simulink model "part7LQR"  (R2022a)
settings: Solver=VariableStepAuto  StartTime=0.0  StopTime=10.0  RelTol=1e-3
settings Model: Creator=HP  LastModifiedBy=HP

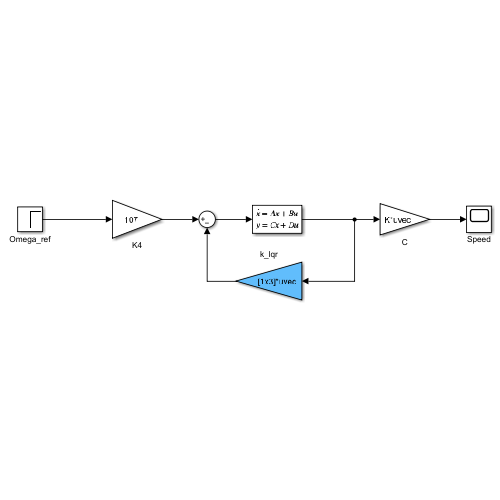
[thumbnail: Simulink's stored preview of the top-level diagram]
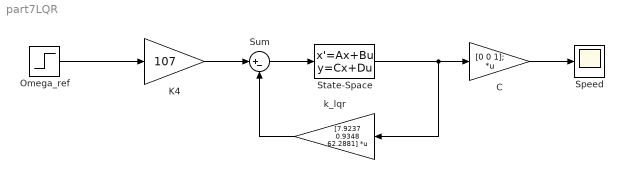
== system part7LQR ==
  C : Gain  Gain=[0 0 1];  Multiplication=Matrix(K*u) (u vector)
  K4 : Gain  Gain=107
  Omega_ref : Step  Time=0  SampleTime=0
  Speed : Scope
  State-Space : StateSpace  A=[-10 0 0;250 -5 -2.5; 0 0.05 -2]  B=[5 0 0]';  C=eye(3)  D=[0 0 0]';  InitialCondition=0
  Sum : Sum  Inputs=|+-
  k_lqr : Gain  Gain="[7.9237 0.9348  62.2881]"  Multiplication=Matrix(K*u) (u vector)
  wires:
  Omega_ref/1 -> K4/1
  K4/1 -> Sum/1
  Sum/1 -> State-Space/1
  k_lqr/1 -> Sum/2
  C/1 -> Speed/1
  State-Space/1 -> C/1, k_lqr/1
